simulink model "A_CruiseControl_Task2"  (R2021b)
settings: Solver=VariableStepAuto  StartTime=0.0  StopTime=400  FixedStep=Ts  RelTol=1e-3
PreLoadFcn:
  | load('CruiseControlTask2_Parameters.mat')
  | load('Parameters.mat')
PostLoadFcn:
  | load('CruiseControlTask2_Parameters.mat')
  | load('Parameters.mat')
StartFcn:
  | load('CruiseControlTask2_Parameters.mat')
undefined symbols (not defined in the file): b, m
CloseFcn:
  | clear
settings Model: Creator=vigne  LastModifiedBy=vigne
settings OptimizationCC: UseDivisionForNetSlopeComputation=on

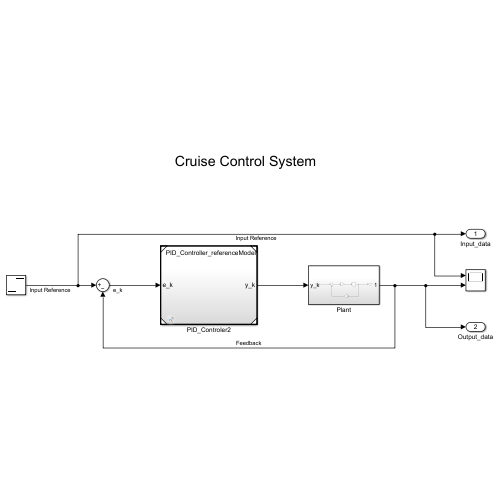
[thumbnail: Simulink's stored preview of the top-level diagram]
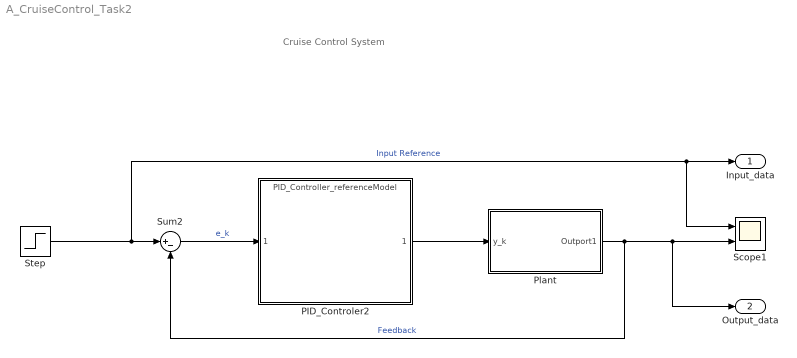
== system A_CruiseControl_Task2 ==
  note: Cruise Control System
  PID_Controler2 : ModelReference  ModelNameDialog=PID_Controller_referenceModel.slx  ModelReferenceVersion=1.16
  Plant : Subsystem
  Scope1 : Scope  NumInputPorts=2
  Step : Step  After=1000  SampleTime=0
  Sum2 : Sum  Inputs=|+-
  Input_data : Outport
  Output_data : Outport  Port=2
  wires:
  PID_Controler2/1 -> Plant/1(y_k)
  Sum2/1 -> PID_Controler2/1  "e_k"
  Step/1 -> Scope1/1, Input_data/1, Sum2/1  "Input Reference"
  Plant/1(Outport1) -> Sum2/2, Output_data/1, Scope1/2  "Feedback"

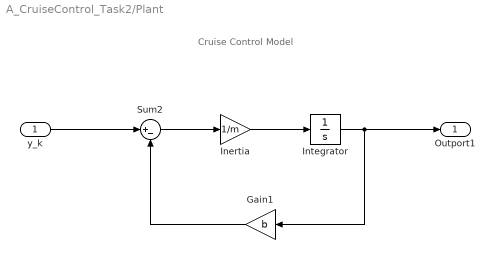
== system A_CruiseControl_Task2/Plant ==
  note: Cruise Control Model
  y_k : Inport
  Gain1 : Gain  Gain=b
  Inertia : Gain  Gain=1/m
  Integrator : Integrator
  Sum2 : Sum  Inputs=|+-
  Outport1 : Outport
  wires:
  Inertia/1 -> Integrator/1
  Integrator/1 -> Outport1/1, Gain1/1
  y_k/1 -> Sum2/1
  Gain1/1 -> Sum2/2
  Sum2/1 -> Inertia/1
